simulink model "mainV02_33"  (R2016b)
settings: Solver=FixedStepAuto  StartTime=0.0  StopTime=inf  FixedStep=Ts  MaxStep=0.2  RelTol=1e-2
undefined symbols (not defined in the file): checks, deltae_degrees, deltafl_degrees, deltafr_degrees, deltar_degrees, deltat_1, deltat_2, deltat_3, deltat_4, deltat_5, Earth, F, ft, groundReaction, initialValues, LD, Light, m, MIL, Newton, Raphson, s, sigbuilder_block, Ts, WGS84
libraries: aerolibutil x19, simulink x17, aerolibtransform2 x7, aerolibasang x4, aerolib6dofsys x4, aerolib6dof2 x4, aerolibwind2 x3, aerolibbdyn x3, aerolibconvert2 x3, aerolibconvert x2, vrlib x2, aerolibatmos2 x1
(part 3 of 5)

== system mainV02_33/Sensors (Feedthrough)/Pitot ==
  Environment : Inport  OutDataTypeStr=Bus: envDataBus
  States : Inport  Port=2  OutDataTypeStr=Bus: plantDataBus
  Bus Selector : BusSelector  OutputSignals=V_body
  Bus Selector1 : BusSelector  OutputSignals=windVelocity
  Sum : Sum  Inputs=|+-
  VaeroMeas_body : Outport
  wires:
  Bus Selector/1 -> Sum/1  "<V_body>"
  States/1 -> Bus Selector/1  "plantData"
  Environment/1 -> Bus Selector1/1
  Bus Selector1/1 -> Sum/2  "<windVelocity>"
  Sum/1 -> VaeroMeas_body/1  "VaeroMeas_body"

== system mainV02_33/Sensors (Feedthrough)/Veleta ==
  States : Inport  OutDataTypeStr=Bus: plantDataBus
  Bus Selector : BusSelector  OutputSignals=alpha,beta
  alphaMeas : Outport
  betaMeas : Outport  Port=2
  wires:
  States/1 -> Bus Selector/1  "plantData"
  Bus Selector/1 -> alphaMeas/1  "<alpha>"
  Bus Selector/2 -> betaMeas/1  "<beta>"

== system mainV02_33/Visualization/Airspeed Indicator ==

== system mainV02_33/Visualization/Altimeter ==

== system mainV02_33/Visualization/Artificial Horizon ==

== system mainV02_33/Visualization/Axes to VR Axes ==
  Xe : Inport
  Concatenate : Concatenate  NumInputs=3
  Constant : Constant  Value=1.01
  Demux : Demux  Outputs=3
  Sum : Sum  Inputs=|++
  rad-->deg : Gain  Gain=-1  SaturateOnIntegerOverflow=on  OutDataTypeStr=Inherit: Same as input  ParamDataTypeStr=Inherit: Same as input
  rad-->deg1 : Gain  Gain=-1  SaturateOnIntegerOverflow=on  OutDataTypeStr=Inherit: Same as input  ParamDataTypeStr=Inherit: Same as input
  Xe VR : Outport
  wires:
  Xe/1 -> Demux/1
  Concatenate/1 -> Xe VR/1
  rad-->deg1/1 -> Concatenate/2
  rad-->deg/1 -> Concatenate/1
  Demux/1 -> Concatenate/3
  Demux/2 -> rad-->deg/1
  Constant/1 -> Sum/2
  Demux/3 -> Sum/1
  Sum/1 -> rad-->deg1/1

== system mainV02_33/Visualization/Climb Rate Indicator ==

== system mainV02_33/Visualization/Euler to VR ==
  Euler Angles : Inport
  Axis Angle Vector : Subsystem
  Constant : Constant  Value=pi/2
  Demux : Demux  Outputs=3
  Mux : Mux  Inputs=2
  Mux1 : Mux  Inputs=2
  Mux2 : Mux  Inputs=2
  Quaternion Multiplication (Pitch & Yaw) : aerolibutil/Quaternion Multiplication
  Quaternion Multiplication (Roll) : aerolibutil/Quaternion Multiplication
  Quaternion Normalization : Subsystem
  Quaternion Normalization1 : Subsystem
  Quaternion Normalization2 : Subsystem
  Sum : Sum  Inputs=|++
  Vr Pitch Axes : Constant  Value=[0 0 1]
  Vr Roll Axes : Constant  Value=[1 0 0]
  Vr Yaw Axes : Constant  Value=[0 -1 0]
  Axis Angle : Outport
  wires:
  Quaternion Multiplication (Roll)/1 -> Axis Angle Vector/1(e0)
  Quaternion Multiplication (Pitch & Yaw)/1 -> Quaternion Multiplication (Roll)/2
  Axis Angle Vector/1(e0_norm) -> Axis Angle/1
  Quaternion Normalization/1(e0_norm) -> Quaternion Multiplication (Roll)/1
  Quaternion Normalization2/1(e0_norm) -> Quaternion Multiplication (Pitch & Yaw)/1
  Quaternion Normalization1/1(e0_norm) -> Quaternion Multiplication (Pitch & Yaw)/2
  Mux2/1 -> Quaternion Normalization2/1(e0)
  Mux1/1 -> Quaternion Normalization1/1(e0)
  Mux/1 -> Quaternion Normalization/1(e0)
  Vr Yaw Axes/1 -> Mux2/2
  Demux/2 -> Mux1/1
  Vr Pitch Axes/1 -> Mux1/2
  Demux/1 -> Mux/1
  Vr Roll Axes/1 -> Mux/2
  Euler Angles/1 -> Demux/1
  Sum/1 -> Mux2/1
  Demux/3 -> Sum/1
  Constant/1 -> Sum/2

== system mainV02_33/Visualization/Heading Indicator ==

== system mainV02_33/Visualization/Subsystem ==
  "X_ned " : Inport
  Euler_angles : Inport  Port=2
  V_body : Inport  Port=3
  V_ned : Inport  Port=4
  Angle Conversion : aerolibconvert2/Angle Conversion  IU=rad  OU=deg
  Angle Conversion1 : aerolibconvert2/Angle Conversion  IU=rad  OU=deg
  Climbrate : Selector  IndexMode=Zero-based  InputPortWidth=3  IndexOptions=Index vector (dialog)  Indices=2  OutputSizes=1
  Concatenate : Concatenate
  Dot Product : DotProduct  SaturateOnIntegerOverflow=on  OutDataTypeStr=Inherit: Inherit via internal rule
  Flightpath Angle : Subsystem
  Heading : Selector  IndexMode=Zero-based  InputPortWidth=3  IndexOptions=Index vector (dialog)  Indices=2  OutputSizes=1
  Height : Selector  IndexMode=Zero-based  InputPortWidth=3  IndexOptions=Index vector (dialog)  Indices=2  OutputSizes=1
  Length Conversion : aerolibconvert2/Length Conversion  IU=m  OU=ft
  Roll Angle : Selector  IndexMode=Zero-based  InputPortWidth=3  IndexOptions=Index vector (dialog)  Indices=0  OutputSizes=1
  Velocity Conversion : aerolibconvert/Velocity Conversion  IU=m/s  OU=kts
  Velocity Conversion1 : aerolibconvert/Velocity Conversion  IU=m/s  OU=ft/s
  rad-->deg1 : Gain  Gain=-1  SaturateOnIntegerOverflow=on  OutDataTypeStr=Inherit: Same as input  ParamDataTypeStr=Inherit: Same as input
  rad-->deg2 : Gain  Gain=-1  SaturateOnIntegerOverflow=on  OutDataTypeStr=Inherit: Same as input  ParamDataTypeStr=Inherit: Same as input
  rad-->deg3 : Gain  Gain=60  SaturateOnIntegerOverflow=on  OutDataTypeStr=Inherit: Same as input  ParamDataTypeStr=Inherit: Same as input
  vt : Sqrt  SaturateOnIntegerOverflow=on
  Airspeed (kts) : Outport
  Height (ft) : Outport  Port=2
  Roll Flightpath (deg) : Outport  Port=3
  Climb Rate (ft/min) : Outport  Port=4
  Heading (deg) : Outport  Port=5
  wires:
  Velocity Conversion1/1 -> rad-->deg3/1
  rad-->deg3/1 -> Climb Rate (ft/min)/1
  V_ned/1 -> Flightpath Angle/1(Ve), Climbrate/1
  Flightpath Angle/1(gamma) -> Concatenate/2
  rad-->deg2/1 -> Velocity Conversion1/1
  Length Conversion/1 -> Height (ft)/1
  Angle Conversion1/1 -> Roll Flightpath (deg)/1
  Height/1 -> rad-->deg1/1
  Angle Conversion/1 -> Heading (deg)/1  "Heading"
  Heading/1 -> Angle Conversion/1
  Velocity Conversion/1 -> Airspeed (kts)/1
  Dot Product/1 -> vt/1
  Roll Angle/1 -> Concatenate/1
  V_body/1 -> Dot Product/2, Dot Product/1
  Concatenate/1 -> Angle Conversion1/1
  vt/1 -> Velocity Conversion/1
  Climbrate/1 -> rad-->deg2/1
  rad-->deg1/1 -> Length Conversion/1
  Euler_angles/1 -> Roll Angle/1, Heading/1
  "X_ned "/1 -> Height/1

== system mainV02_33/Environment/Terrain/Reaction ==
  X : Inport
  V : Inport  Port=2
  -D1 : Gain  Gain=-groundReaction.D
  -K2 : Gain  Gain=-groundReaction.K
  Constant3 : Constant  Value=0
  Constant4 : Constant  Value=0
  Constant5 : Constant  Value=0
  Mux1 : Mux  Inputs=3
  Product1 : Product
  Sel5 : Selector  InputPortWidth=3  IndexOptions=Index vector (dialog)  Indices=3  OutputSizes=1
  Sel6 : Selector  InputPortWidth=3  IndexOptions=Index vector (dialog)  Indices=3  OutputSizes=1
  Sqrt1 : Sqrt  SaturateOnIntegerOverflow=on
  Sum4 : Sum  Inputs=|++
  Sum5 : Sum  Inputs=-+
  Switch3 : Switch  Criteria=u2 > Threshold
  Ze2height1 : UnaryMinus
  Ze_dot2height_dot3 : UnaryMinus
  height2d2 : UnaryMinus
  height2d3 : UnaryMinus
  hground_value1 : Constant  Value=initialValues.href  OutDataTypeStr=double
  hground1 : Outport  Unit=m
  F_earth : Outport  Port=2
  wires:
  Ze2height1/1 -> Sum5/2  "alt"
  X/1 -> Sel6/1
  Sel6/1 -> Ze2height1/1
  Sel5/1 -> Ze_dot2height_dot3/1
  hground_value1/1 -> Sum5/1
  Constant3/1 -> Switch3/1
  Switch3/1 -> height2d2/1
  height2d2/1 -> Sqrt1/1  "d"
  -K2/1 -> Sum4/1
  Product1/1 -> height2d3/1
  height2d3/1 -> Mux1/3
  Sum5/1 -> hground1/1, -K2/1, Switch3/3, Switch3/2  "z"
  Sqrt1/1 -> Product1/1
  Ze_dot2height_dot3/1 -> -D1/1  "z_dot"
  -D1/1 -> Sum4/2
  Sum4/1 -> Product1/2
  V/1 -> Sel5/1
  Mux1/1 -> F_earth/1  "F_earth"
  Constant5/1 -> Mux1/2
  Constant4/1 -> Mux1/1

== system mainV02_33/Environment/Terrain/Reaction1 ==
  X : Inport
  V : Inport  Port=2
  -D1 : Gain  Gain=-groundReaction.D
  -K2 : Gain  Gain=-groundReaction.K
  Constant3 : Constant  Value=0
  Constant4 : Constant  Value=0
  Constant5 : Constant  Value=0
  Mux1 : Mux  Inputs=3
  Product1 : Product
  Sel5 : Selector  InputPortWidth=3  IndexOptions=Index vector (dialog)  Indices=3  OutputSizes=1
  Sel6 : Selector  InputPortWidth=3  IndexOptions=Index vector (dialog)  Indices=3  OutputSizes=1
  Sqrt1 : Sqrt  SaturateOnIntegerOverflow=on
  Sum4 : Sum  Inputs=|++
  Sum5 : Sum  Inputs=-+
  Switch3 : Switch  Criteria=u2 > Threshold
  Ze2height1 : UnaryMinus
  Ze_dot2height_dot3 : UnaryMinus
  height2d2 : UnaryMinus
  height2d3 : UnaryMinus
  hground_value1 : Constant  Value=initialValues.href  OutDataTypeStr=double
  hground1 : Outport  Unit=m
  F_earth : Outport  Port=2
  wires:
  Ze2height1/1 -> Sum5/2  "alt"
  X/1 -> Sel6/1
  Sel6/1 -> Ze2height1/1
  Sel5/1 -> Ze_dot2height_dot3/1
  hground_value1/1 -> Sum5/1
  Constant3/1 -> Switch3/1
  Switch3/1 -> height2d2/1
  height2d2/1 -> Sqrt1/1  "d"
  -K2/1 -> Sum4/1
  Product1/1 -> height2d3/1
  height2d3/1 -> Mux1/3
  Sum5/1 -> hground1/1, -K2/1, Switch3/3, Switch3/2  "z"
  Sqrt1/1 -> Product1/1
  Ze_dot2height_dot3/1 -> -D1/1  "z_dot"
  -D1/1 -> Sum4/2
  Sum4/1 -> Product1/2
  V/1 -> Sel5/1
  Mux1/1 -> F_earth/1  "F_earth"
  Constant5/1 -> Mux1/2
  Constant4/1 -> Mux1/1

== system mainV02_33/Environment/Terrain/Reaction2 ==
  X : Inport
  V : Inport  Port=2
  -D1 : Gain  Gain=-groundReaction.D
  -K2 : Gain  Gain=-groundReaction.K
  Constant3 : Constant  Value=0
  Constant4 : Constant  Value=0
  Constant5 : Constant  Value=0
  Mux1 : Mux  Inputs=3
  Product1 : Product
  Sel5 : Selector  InputPortWidth=3  IndexOptions=Index vector (dialog)  Indices=3  OutputSizes=1
  Sel6 : Selector  InputPortWidth=3  IndexOptions=Index vector (dialog)  Indices=3  OutputSizes=1
  Sqrt1 : Sqrt  SaturateOnIntegerOverflow=on
  Sum4 : Sum  Inputs=|++
  Sum5 : Sum  Inputs=-+
  Switch3 : Switch  Criteria=u2 > Threshold
  Ze2height1 : UnaryMinus
  Ze_dot2height_dot3 : UnaryMinus
  height2d2 : UnaryMinus
  height2d3 : UnaryMinus
  hground_value1 : Constant  Value=initialValues.href  OutDataTypeStr=double
  hground1 : Outport  Unit=m
  F_earth : Outport  Port=2
  wires:
  Ze2height1/1 -> Sum5/2  "alt"
  X/1 -> Sel6/1
  Sel6/1 -> Ze2height1/1
  Sel5/1 -> Ze_dot2height_dot3/1
  hground_value1/1 -> Sum5/1
  Constant3/1 -> Switch3/1
  Switch3/1 -> height2d2/1
  height2d2/1 -> Sqrt1/1  "d"
  -K2/1 -> Sum4/1
  Product1/1 -> height2d3/1
  height2d3/1 -> Mux1/3
  Sum5/1 -> hground1/1, -K2/1, Switch3/3, Switch3/2  "z"
  Sqrt1/1 -> Product1/1
  Ze_dot2height_dot3/1 -> -D1/1  "z_dot"
  -D1/1 -> Sum4/2
  Sum4/1 -> Product1/2
  V/1 -> Sel5/1
  Mux1/1 -> F_earth/1  "F_earth"
  Constant5/1 -> Mux1/2
  Constant4/1 -> Mux1/1

== system mainV02_33/FCS/Quad actuator commands/Altitude ==
  Altitude cmd : Inport
  Bias : Bias  Bias=LD.FCS.Quadcopter.Throttle.bias
  dThrottle : Gain  Gain=LD.FCS.Quadcopter.Throttle.dThrottle
  T5 : Outport
  T3 : Outport  Port=2
  T4 : Outport  Port=3
  T2 : Outport  Port=4
  wires:
  Bias/1 -> T5/1, T4/1, T3/1, T2/1
  Altitude cmd/1 -> dThrottle/1
  dThrottle/1 -> Bias/1

== system mainV02_33/FCS/Quad actuator commands/Pitch ==
  Pitch Cmd : Inport
  Constant1 : Constant  Value=LD.Inertia.CG
  Constant2 : Constant  Value=LD.Inertia.CG
  Divide : Product  Inputs=*/
  Product : Product
  Product1 : Product
  Selector : Selector  InputPortWidth=3  IndexOptions=Index vector (dialog)  Indices=1  OutputSizes=1
  Selector1 : Selector  InputPortWidth=3  IndexOptions=Index vector (dialog)  Indices=1  OutputSizes=1
  Sum1 : Sum  Inputs=+-|
  Sum2 : Sum  Inputs=+-|
  dPitch : Gain  Gain=LD.FCS.Quadcopter.Pitch.dPitch
  "motor2 position " : Constant  Value=LD.Propulsion.motor2.Position
  motor2 position 1 : Constant  Value=LD.Propulsion.motor3.Position
  T5 : Outport
  T3 : Outport  Port=2
  T2 : Outport  Port=3
  T4 : Outport  Port=4
  wires:
  Pitch Cmd/1 -> dPitch/1
  Product/1 -> T3/1
  dPitch/1 -> T5/1, Product1/1, Product/1, T2/1
  Constant1/1 -> Sum1/2
  "motor2 position "/1 -> Sum1/1
  Sum1/1 -> Selector/1  "arm"
  Constant2/1 -> Sum2/2
  motor2 position 1/1 -> Sum2/1
  Sum2/1 -> Selector1/1  "arm"
  Selector/1 -> Divide/1
  Selector1/1 -> Divide/2
  Product1/1 -> T4/1
  [Gain] -> Product/2
  [Gain] -> Product1/2
  Divide/1 -> [Gain]

== system mainV02_33/FCS/Quad actuator commands/Roll ==
  Roll Cmd : Inport
  Gain : Gain  Gain=-1
  Gain1 : Gain  Gain=-1
  dRoll : Gain  Gain=LD.FCS.Quadcopter.Roll.dRoll
  T4 : Outport
  T2 : Outport  Port=2
  T5 : Outport  Port=3
  T3 : Outport  Port=4
  wires:
  Gain/1 -> T2/1
  dRoll/1 -> Gain1/1, Gain/1, T4/1, T5/1
  Roll Cmd/1 -> dRoll/1
  Gain1/1 -> T3/1

== system mainV02_33/FCS/Quad actuator commands/Yaw ==
  Yaw Cmd : Inport
  Gain : Gain  Gain=-1
  Gain1 : Gain  Gain=-1
  dYaw : Gain  Gain=LD.FCS.Quadcopter.Yaw.dYaw
  T5 : Outport
  T4 : Outport  Port=2
  T3 : Outport  Port=3
  T2 : Outport  Port=4
  wires:
  Yaw Cmd/1 -> dYaw/1
  dYaw/1 -> Gain1/1, T4/1, T2/1, Gain/1
  Gain1/1 -> T5/1
  Gain/1 -> T3/1

== system mainV02_33/LIBIS Plant/Aerodynamics/CD ==
  prelook-ups : Inport
  plantData : Inport  Port=2
  actuators : Inport  Port=3
  Add : Sum  Inputs=+++++++
  Bus Selector : BusSelector  OutputSignals=alpha,alpha_dot,Omega_body.q
  Bus Selector1 : BusSelector  OutputSignals=alpha,beta,alt,xcg,deltae,deltar,deltafr,deltafl
  Bus Selector2 : BusSelector  OutputSignals=deltae,deltafr,deltafl
  CD0 : Interpolation_n-D  NumberOfTableDimensions=8  Table=LD.Stability.CD0  ExtrapMethod=Clip  DiagnosticForOutOfRangeInput=Warning  RequireIndexFractionAsBus=on  ValidIndexMayReachLast=on  InternalRulePriority=Speed
      settings: InputPortMap=u0,u1,u2,u3,u4,u5,u6,u7
  CDalpha : Interpolation_n-D  NumberOfTableDimensions=8  Table=LD.Stability.CDalpha  ExtrapMethod=Clip  DiagnosticForOutOfRangeInput=Warning  RequireIndexFractionAsBus=on  ValidIndexMayReachLast=on  InternalRulePriority=Speed
      settings: InputPortMap=u0,u1,u2,u3,u4,u5,u6,u7
  CDalpha_dot : Interpolation_n-D  NumberOfTableDimensions=8  Table=LD.Stability.CDalpha_dot  ExtrapMethod=Clip  RequireIndexFractionAsBus=on  ValidIndexMayReachLast=on  InternalRulePriority=Speed
      settings: InputPortMap=u0,u1,u2,u3,u4,u5,u6,u7
  CDdeltae : Interpolation_n-D  NumberOfTableDimensions=8  Table=LD.Stability.CDdeltae  ExtrapMethod=Clip  RequireIndexFractionAsBus=on  ValidIndexMayReachLast=on  InternalRulePriority=Speed
      settings: InputPortMap=u0,u1,u2,u3,u4,u5,u6,u7
  CDdeltafr : Interpolation_n-D  NumberOfTableDimensions=8  Table=LD.Stability.CDdeltafr  ExtrapMethod=Clip  RequireIndexFractionAsBus=on  ValidIndexMayReachLast=on  InternalRulePriority=Speed
      settings: InputPortMap=u0,u1,u2,u3,u4,u5,u6,u7
  CDdeltafrl : Interpolation_n-D  NumberOfTableDimensions=8  Table=LD.Stability.CDdeltafl  ExtrapMethod=Clip  RequireIndexFractionAsBus=on  ValidIndexMayReachLast=on  InternalRulePriority=Speed
      settings: InputPortMap=u0,u1,u2,u3,u4,u5,u6,u7
  CDq : Interpolation_n-D  NumberOfTableDimensions=8  Table=LD.Stability.CDq  ExtrapMethod=Clip  RequireIndexFractionAsBus=on  ValidIndexMayReachLast=on  InternalRulePriority=Speed
      settings: InputPortMap=u0,u1,u2,u3,u4,u5,u6,u7
  Product{,1..5} (6 alike) : Product
  CD : Outport
  wires:
  prelook-ups/1 -> Bus Selector1/1
  CD0/1 -> Add/1
  Add/1 -> CD/1
  plantData/1 -> Bus Selector/1
  actuators/1 -> Bus Selector2/1
  Product/1 -> Add/2
  Bus Selector/1 -> Product/2  "<alpha>"
  Bus Selector2/1 -> Product3/2  "<deltae>"
  CDdeltae/1 -> Product3/1
  Product3/1 -> Add/5
  Product2/1 -> Add/4
  Product1/1 -> Add/3
  CDalpha_dot/1 -> Product1/1
  CDq/1 -> Product2/1
  Bus Selector/3 -> Product2/2  "<q>"
  Bus Selector/2 -> Product1/2  "<alpha_dot>"
  Bus Selector1/8 -> CD0/8, CDalpha/8, CDq/8, CDdeltafrl/8, CDdeltafr/8, CDdeltae/8, CDalpha_dot/8  "<deltafl>"
  Bus Selector1/7 -> CD0/7, CDalpha/7, CDq/7, CDdeltafrl/7, CDdeltafr/7, CDdeltae/7, CDalpha_dot/7  "<deltafr>"
  Bus Selector1/6 -> CD0/6, CDalpha/6, CDq/6, CDdeltafrl/6, CDdeltafr/6, CDdeltae/6, CDalpha_dot/6  "<deltar>"
  Bus Selector1/5 -> CD0/5, CDalpha/5, CDq/5, CDdeltafrl/5, CDdeltafr/5, CDdeltae/5, CDalpha_dot/5  "<deltae>"
  Bus Selector1/3 -> CD0/3, CDalpha/3, CDq/3, CDdeltafrl/3, CDdeltafr/3, CDdeltae/3, CDalpha_dot/3  "<alt>"
  Bus Selector1/4 -> CD0/4, CDalpha/4, CDq/4, CDdeltafrl/4, CDdeltafr/4, CDdeltae/4, CDalpha_dot/4  "<xcg>"
  Bus Selector1/1 -> CD0/1, CDalpha/1, CDdeltafrl/1, CDdeltafr/1, CDdeltae/1, CDq/1, CDalpha_dot/1  "<alpha>"
  Bus Selector2/3 -> Product5/2  "<deltafl>"
  CDdeltafrl/1 -> Product5/1
  Product5/1 -> Add/7
  Product4/1 -> Add/6
  CDdeltafr/1 -> Product4/1
  Bus Selector2/2 -> Product4/2  "<deltafr>"
  Bus Selector1/2 -> CD0/2, CDdeltafrl/2, CDdeltafr/2, CDdeltae/2, CDq/2, CDalpha_dot/2, CDalpha/2  "<beta>"
  CDalpha/1 -> Product/1

== system mainV02_33/LIBIS Plant/Aerodynamics/CL ==
  prelook-ups : Inport
  plantData : Inport  Port=2
  actuators : Inport  Port=3
  Add1 : Sum  Inputs=+++++++
  Bus Selector2 : BusSelector  OutputSignals=alpha,alpha_dot,Omega_body.q
  Bus Selector4 : BusSelector  OutputSignals=alpha,beta,alt,xcg,deltae,deltar,deltafr,deltafl
  Bus Selector5 : BusSelector  OutputSignals=deltae,deltafr,deltafl
  CL0 : Interpolation_n-D  NumberOfTableDimensions=8  Table=LD.Stability.CL0  RequireIndexFractionAsBus=on  InternalRulePriority=Speed
      settings: InputPortMap=u0,u1,u2,u3,u4,u5,u6,u7
  CLalpha : Interpolation_n-D  NumberOfTableDimensions=8  Table=LD.Stability.CLalpha  ExtrapMethod=Clip  DiagnosticForOutOfRangeInput=Warning  RequireIndexFractionAsBus=on  ValidIndexMayReachLast=on  InternalRulePriority=Speed
      settings: InputPortMap=u0,u1,u2,u3,u4,u5,u6,u7
  CLalpha_dot : Interpolation_n-D  NumberOfTableDimensions=8  Table=LD.Stability.CLalpha_dot  ExtrapMethod=Clip  RequireIndexFractionAsBus=on  ValidIndexMayReachLast=on  InternalRulePriority=Speed
      settings: InputPortMap=u0,u1,u2,u3,u4,u5,u6,u7
  CLdeltae : Interpolation_n-D  NumberOfTableDimensions=8  Table=LD.Stability.CLdeltae  ExtrapMethod=Clip  RequireIndexFractionAsBus=on  ValidIndexMayReachLast=on  InternalRulePriority=Speed
      settings: InputPortMap=u0,u1,u2,u3,u4,u5,u6,u7
  CLdeltafr : Interpolation_n-D  NumberOfTableDimensions=8  Table=LD.Stability.CLdeltafr  ExtrapMethod=Clip  RequireIndexFractionAsBus=on  ValidIndexMayReachLast=on  InternalRulePriority=Speed
      settings: InputPortMap=u0,u1,u2,u3,u4,u5,u6,u7
  CLdeltafrl : Interpolation_n-D  NumberOfTableDimensions=8  Table=LD.Stability.CLdeltafl  ExtrapMethod=Clip  RequireIndexFractionAsBus=on  ValidIndexMayReachLast=on  InternalRulePriority=Speed
      settings: InputPortMap=u0,u1,u2,u3,u4,u5,u6,u7
  CLq : Interpolation_n-D  NumberOfTableDimensions=8  Table=LD.Stability.CLq  ExtrapMethod=Clip  RequireIndexFractionAsBus=on  ValidIndexMayReachLast=on  InternalRulePriority=Speed
      settings: InputPortMap=u0,u1,u2,u3,u4,u5,u6,u7
  Product{6..11} (6 alike) : Product
  CL : Outport
  wires:
  prelook-ups/1 -> Bus Selector4/1
  CL0/1 -> Add1/1
  Add1/1 -> CL/1
  plantData/1 -> Bus Selector2/1
  actuators/1 -> Bus Selector5/1
  Product6/1 -> Add1/2
  Bus Selector2/1 -> Product6/2  "<alpha>"
  Bus Selector5/1 -> Product9/2  "<deltae>"
  CLdeltae/1 -> Product9/1
  Product9/1 -> Add1/5
  Product8/1 -> Add1/4
  Product7/1 -> Add1/3
  CLalpha_dot/1 -> Product7/1
  CLq/1 -> Product8/1
  Bus Selector2/3 -> Product8/2  "<q>"
  Bus Selector2/2 -> Product7/2  "<alpha_dot>"
  Bus Selector4/8 -> CL0/8, CLalpha/8, CLq/8, CLdeltafrl/8, CLdeltafr/8, CLdeltae/8, CLalpha_dot/8  "<deltafl>"
  Bus Selector4/7 -> CL0/7, CLalpha/7, CLq/7, CLdeltafrl/7, CLdeltafr/7, CLdeltae/7, CLalpha_dot/7  "<deltafr>"
  Bus Selector4/6 -> CL0/6, CLalpha/6, CLq/6, CLdeltafrl/6, CLdeltafr/6, CLdeltae/6, CLalpha_dot/6  "<deltar>"
  Bus Selector4/5 -> CL0/5, CLalpha/5, CLq/5, CLdeltafrl/5, CLdeltafr/5, CLdeltae/5, CLalpha_dot/5  "<deltae>"
  Bus Selector4/3 -> CL0/3, CLalpha/3, CLq/3, CLdeltafrl/3, CLdeltafr/3, CLdeltae/3, CLalpha_dot/3  "<alt>"
  Bus Selector4/4 -> CL0/4, CLalpha/4, CLq/4, CLdeltafrl/4, CLdeltafr/4, CLdeltae/4, CLalpha_dot/4  "<xcg>"
  Bus Selector4/1 -> CL0/1, CLalpha/1, CLdeltafrl/1, CLdeltafr/1, CLdeltae/1, CLq/1, CLalpha_dot/1  "<alpha>"
  Bus Selector5/3 -> Product11/2  "<deltafl>"
  CLdeltafrl/1 -> Product11/1
  Product11/1 -> Add1/7
  Product10/1 -> Add1/6
  CLdeltafr/1 -> Product10/1
  Bus Selector5/2 -> Product10/2  "<deltafr>"
  Bus Selector4/2 -> CL0/2, CLdeltafrl/2, CLdeltafr/2, CLdeltae/2, CLq/2, CLalpha_dot/2, CLalpha/2  "<beta>"
  CLalpha/1 -> Product6/1

== system mainV02_33/LIBIS Plant/Aerodynamics/CY ==
  prelook-ups : Inport
  plantData : Inport  Port=2
  actuators : Inport  Port=3
  Add : Sum  Inputs=++++++
  Bus Selector : BusSelector  OutputSignals=beta,Omega_body.p,Omega_body.r
  Bus Selector1 : BusSelector  OutputSignals=alpha,beta,alt,xcg,deltae,deltar,deltafr,deltafl
  Bus Selector2 : BusSelector  OutputSignals=deltar,deltafr,deltafl
  CYbeta : Interpolation_n-D  NumberOfTableDimensions=8  Table=LD.Stability.CYbeta  ExtrapMethod=Clip  RequireIndexFractionAsBus=on  ValidIndexMayReachLast=on  InternalRulePriority=Speed
      settings: InputPortMap=u0,u1,u2,u3,u4,u5,u6,u7
  CYdeltafl : Interpolation_n-D  NumberOfTableDimensions=8  Table=LD.Stability.CYdeltafl  ExtrapMethod=Clip  RequireIndexFractionAsBus=on  ValidIndexMayReachLast=on  InternalRulePriority=Speed
      settings: InputPortMap=u0,u1,u2,u3,u4,u5,u6,u7
  CYdeltafr : Interpolation_n-D  NumberOfTableDimensions=8  Table=LD.Stability.CYdeltafr  ExtrapMethod=Clip  RequireIndexFractionAsBus=on  ValidIndexMayReachLast=on  InternalRulePriority=Speed
      settings: InputPortMap=u0,u1,u2,u3,u4,u5,u6,u7
  "CYdeltar " : Interpolation_n-D  NumberOfTableDimensions=8  Table=LD.Stability.CYdeltar  ExtrapMethod=Clip  RequireIndexFractionAsBus=on  ValidIndexMayReachLast=on  InternalRulePriority=Speed
      settings: InputPortMap=u0,u1,u2,u3,u4,u5,u6,u7
  CYp : Interpolation_n-D  NumberOfTableDimensions=8  Table=LD.Stability.CYp  ExtrapMethod=Clip  RequireIndexFractionAsBus=on  ValidIndexMayReachLast=on  InternalRulePriority=Speed
      settings: InputPortMap=u0,u1,u2,u3,u4,u5,u6,u7
  CYr : Interpolation_n-D  NumberOfTableDimensions=8  Table=LD.Stability.CYr  ExtrapMethod=Clip  RequireIndexFractionAsBus=on  ValidIndexMayReachLast=on  InternalRulePriority=Speed
      settings: InputPortMap=u0,u1,u2,u3,u4,u5,u6,u7
  Product{,1..5} (6 alike) : Product
  CY : Outport
  wires:
  Bus Selector1/8 -> CYbeta/8, CYr/8, "CYdeltar "/8, CYdeltafl/8, CYdeltafr/8, CYp/8  "<deltafl>"
  Bus Selector1/7 -> CYbeta/7, CYr/7, "CYdeltar "/7, CYdeltafl/7, CYdeltafr/7, CYp/7  "<deltafr>"
  Bus Selector1/6 -> CYbeta/6, CYr/6, "CYdeltar "/6, CYdeltafl/6, CYdeltafr/6, CYp/6  "<deltar>"
  prelook-ups/1 -> Bus Selector1/1
  Bus Selector1/5 -> CYbeta/5, CYr/5, "CYdeltar "/5, CYdeltafl/5, CYdeltafr/5, CYp/5  "<deltae>"
  Bus Selector1/3 -> CYbeta/3, CYr/3, "CYdeltar "/3, CYdeltafl/3, CYdeltafr/3, CYp/3  "<alt>"
  Bus Selector1/4 -> CYbeta/4, CYr/4, "CYdeltar "/4, CYdeltafl/4, CYdeltafr/4, CYp/4  "<xcg>"
  Bus Selector1/1 -> CYbeta/1, CYdeltafl/1, CYdeltafr/1, "CYdeltar "/1, CYr/1, CYp/1  "<alpha>"
  Add/1 -> CY/1
  plantData/1 -> Bus Selector/1
  actuators/1 -> Bus Selector2/1
  CYbeta/1 -> Product/1
  Product/1 -> Add/1
  Bus Selector/1 -> Product/2  "<beta>"
  Bus Selector2/1 -> Product3/2  "<deltar>"
  "CYdeltar "/1 -> Product3/1
  Product3/1 -> Add/4
  Product2/1 -> Add/3
  Product1/1 -> Add/2
  CYp/1 -> Product1/1
  CYr/1 -> Product2/1
  Bus Selector/3 -> Product2/2  "<r>"
  Bus Selector/2 -> Product1/2  "<p>"
  CYdeltafl/1 -> Product5/1
  Product5/1 -> Add/6
  Product4/1 -> Add/5
  CYdeltafr/1 -> Product4/1
  Bus Selector2/2 -> Product4/2  "<deltafr>"
  Bus Selector2/3 -> Product5/2  "<deltafl>"
  Bus Selector1/2 -> CYdeltafl/2, CYdeltafr/2, "CYdeltar "/2, CYr/2, CYp/2, CYbeta/2  "<beta>"

== system mainV02_33/LIBIS Plant/Aerodynamics/Cl ==
  prelook-ups1 : Inport
  plantData : Inport  Port=2
  actuators : Inport  Port=3
  Add1 : Sum  Inputs=++++++
  Bus Selector3 : BusSelector  OutputSignals=beta,Omega_body.p,Omega_body.r
  Bus Selector4 : BusSelector  OutputSignals=alpha,beta,alt,xcg,deltae,deltar,deltafr,deltafl
  Bus Selector5 : BusSelector  OutputSignals=deltar,deltafr,deltafl
  Clbeta : Interpolation_n-D  NumberOfTableDimensions=8  Table=LD.Stability.Clbeta  ExtrapMethod=Clip  RequireIndexFractionAsBus=on  ValidIndexMayReachLast=on  InternalRulePriority=Speed
      settings: InputPortMap=u0,u1,u2,u3,u4,u5,u6,u7
  Cldeltafl : Interpolation_n-D  NumberOfTableDimensions=8  Table=LD.Stability.Cldeltafl  ExtrapMethod=Clip  RequireIndexFractionAsBus=on  ValidIndexMayReachLast=on  InternalRulePriority=Speed
      settings: InputPortMap=u0,u1,u2,u3,u4,u5,u6,u7
  Cldeltafr : Interpolation_n-D  NumberOfTableDimensions=8  Table=LD.Stability.Cldeltafr  ExtrapMethod=Clip  RequireIndexFractionAsBus=on  ValidIndexMayReachLast=on  InternalRulePriority=Speed
      settings: InputPortMap=u0,u1,u2,u3,u4,u5,u6,u7
  "Cldeltar " : Interpolation_n-D  NumberOfTableDimensions=8  Table=LD.Stability.Cldeltar  ExtrapMethod=Clip  RequireIndexFractionAsBus=on  ValidIndexMayReachLast=on  InternalRulePriority=Speed
      settings: InputPortMap=u0,u1,u2,u3,u4,u5,u6,u7
  Clp : Interpolation_n-D  NumberOfTableDimensions=8  Table=LD.Stability.Clp  ExtrapMethod=Clip  RequireIndexFractionAsBus=on  ValidIndexMayReachLast=on  InternalRulePriority=Speed
      settings: InputPortMap=u0,u1,u2,u3,u4,u5,u6,u7
  Clr : Interpolation_n-D  NumberOfTableDimensions=8  Table=LD.Stability.Clr  ExtrapMethod=Clip  RequireIndexFractionAsBus=on  ValidIndexMayReachLast=on  InternalRulePriority=Speed
      settings: InputPortMap=u0,u1,u2,u3,u4,u5,u6,u7
  Product{6..11} (6 alike) : Product
  Cl : Outport
  wires:
  Bus Selector4/8 -> Clbeta/8, Clr/8, "Cldeltar "/8, Cldeltafl/8, Cldeltafr/8, Clp/8  "<deltafl>"
  Bus Selector4/7 -> Clbeta/7, Clr/7, "Cldeltar "/7, Cldeltafl/7, Cldeltafr/7, Clp/7  "<deltafr>"
  Bus Selector4/6 -> Clbeta/6, Clr/6, "Cldeltar "/6, Cldeltafl/6, Cldeltafr/6, Clp/6  "<deltar>"
  prelook-ups1/1 -> Bus Selector4/1
  Bus Selector4/5 -> Clbeta/5, Clr/5, "Cldeltar "/5, Cldeltafl/5, Cldeltafr/5, Clp/5  "<deltae>"
  Bus Selector4/3 -> Clbeta/3, Clr/3, "Cldeltar "/3, Cldeltafl/3, Cldeltafr/3, Clp/3  "<alt>"
  Bus Selector4/4 -> Clbeta/4, Clr/4, "Cldeltar "/4, Cldeltafl/4, Cldeltafr/4, Clp/4  "<xcg>"
  Bus Selector4/1 -> Clbeta/1, Cldeltafl/1, Cldeltafr/1, "Cldeltar "/1, Clr/1, Clp/1  "<alpha>"
  Add1/1 -> Cl/1
  plantData/1 -> Bus Selector3/1
  actuators/1 -> Bus Selector5/1
  Clbeta/1 -> Product6/1
  Product6/1 -> Add1/1
  Bus Selector3/1 -> Product6/2  "<beta>"
  Bus Selector5/1 -> Product9/2  "<deltar>"
  "Cldeltar "/1 -> Product9/1
  Product9/1 -> Add1/4
  Product8/1 -> Add1/3
  Product7/1 -> Add1/2
  Clp/1 -> Product7/1
  Clr/1 -> Product8/1
  Bus Selector3/3 -> Product8/2  "<r>"
  Bus Selector3/2 -> Product7/2  "<p>"
  Cldeltafl/1 -> Product11/1
  Product11/1 -> Add1/6
  Product10/1 -> Add1/5
  Cldeltafr/1 -> Product10/1
  Bus Selector5/2 -> Product10/2  "<deltafr>"
  Bus Selector5/3 -> Product11/2  "<deltafl>"
  Bus Selector4/2 -> Cldeltafl/2, Cldeltafr/2, "Cldeltar "/2, Clr/2, Clp/2, Clbeta/2  "<beta>"

== system mainV02_33/LIBIS Plant/Aerodynamics/Cm ==
  prelook-ups : Inport
  plantData : Inport  Port=2
  actuators : Inport  Port=3
  Add2 : Sum  Inputs=+++++++
  Bus Selector2 : BusSelector  OutputSignals=alpha,alpha_dot,Omega_body.q
  Bus Selector4 : BusSelector  OutputSignals=alpha,beta,alt,xcg,deltae,deltar,deltafr,deltafl
  Bus Selector5 : BusSelector  OutputSignals=deltae,deltafr,deltafl
  Cm0 : Interpolation_n-D  NumberOfTableDimensions=8  Table=LD.Stability.Cm0  RequireIndexFractionAsBus=on  InternalRulePriority=Speed
      settings: InputPortMap=u0,u1,u2,u3,u4,u5,u6,u7
  Cmalpha : Interpolation_n-D  NumberOfTableDimensions=8  Table=LD.Stability.Cmalpha  ExtrapMethod=Clip  RequireIndexFractionAsBus=on  ValidIndexMayReachLast=on  InternalRulePriority=Speed
      settings: InputPortMap=u0,u1,u2,u3,u4,u5,u6,u7
  Cmalpha_dot : Interpolation_n-D  NumberOfTableDimensions=8  Table=LD.Stability.Cmalpha_dot  ExtrapMethod=Clip  RequireIndexFractionAsBus=on  ValidIndexMayReachLast=on  InternalRulePriority=Speed
      settings: InputPortMap=u0,u1,u2,u3,u4,u5,u6,u7
  Cmdeltae : Interpolation_n-D  NumberOfTableDimensions=8  Table=LD.Stability.Cmdeltae  ExtrapMethod=Clip  RequireIndexFractionAsBus=on  ValidIndexMayReachLast=on  InternalRulePriority=Speed
      settings: InputPortMap=u0,u1,u2,u3,u4,u5,u6,u7
  Cmdeltafl : Interpolation_n-D  NumberOfTableDimensions=8  Table=LD.Stability.CLdeltafl  ExtrapMethod=Clip  RequireIndexFractionAsBus=on  ValidIndexMayReachLast=on  InternalRulePriority=Speed
      settings: InputPortMap=u0,u1,u2,u3,u4,u5,u6,u7
  Cmdeltafr : Interpolation_n-D  NumberOfTableDimensions=8  Table=LD.Stability.Cmdeltafr  ExtrapMethod=Clip  RequireIndexFractionAsBus=on  ValidIndexMayReachLast=on  InternalRulePriority=Speed
      settings: InputPortMap=u0,u1,u2,u3,u4,u5,u6,u7
  Cmq : Interpolation_n-D  NumberOfTableDimensions=8  Table=LD.Stability.Cmq  ExtrapMethod=Clip  RequireIndexFractionAsBus=on  ValidIndexMayReachLast=on  InternalRulePriority=Speed
      settings: InputPortMap=u0,u1,u2,u3,u4,u5,u6,u7
  Product{6..11} (6 alike) : Product
  Cm : Outport
  wires:
  prelook-ups/1 -> Bus Selector4/1
  Cm0/1 -> Add2/1
  Add2/1 -> Cm/1
  plantData/1 -> Bus Selector2/1
  actuators/1 -> Bus Selector5/1
  Product6/1 -> Add2/2
  Bus Selector2/1 -> Product6/2  "<alpha>"
  Bus Selector5/1 -> Product9/2  "<deltae>"
  Cmdeltae/1 -> Product9/1
  Product9/1 -> Add2/5
  Product8/1 -> Add2/4
  Product7/1 -> Add2/3
  Cmalpha_dot/1 -> Product7/1
  Cmq/1 -> Product8/1
  Bus Selector2/3 -> Product8/2  "<q>"
  Bus Selector2/2 -> Product7/2  "<alpha_dot>"
  Bus Selector4/8 -> Cm0/8, Cmalpha/8, Cmq/8, Cmdeltafl/8, Cmdeltafr/8, Cmdeltae/8, Cmalpha_dot/8  "<deltafl>"
  Bus Selector4/7 -> Cm0/7, Cmalpha/7, Cmq/7, Cmdeltafl/7, Cmdeltafr/7, Cmdeltae/7, Cmalpha_dot/7  "<deltafr>"
  Bus Selector4/6 -> Cm0/6, Cmalpha/6, Cmq/6, Cmdeltafl/6, Cmdeltafr/6, Cmdeltae/6, Cmalpha_dot/6  "<deltar>"
  Bus Selector4/5 -> Cm0/5, Cmalpha/5, Cmq/5, Cmdeltafl/5, Cmdeltafr/5, Cmdeltae/5, Cmalpha_dot/5  "<deltae>"
  Bus Selector4/3 -> Cm0/3, Cmalpha/3, Cmq/3, Cmdeltafl/3, Cmdeltafr/3, Cmdeltae/3, Cmalpha_dot/3  "<alt>"
  Bus Selector4/4 -> Cm0/4, Cmalpha/4, Cmq/4, Cmdeltafl/4, Cmdeltafr/4, Cmdeltae/4, Cmalpha_dot/4  "<xcg>"
  Bus Selector4/1 -> Cm0/1, Cmalpha/1, Cmdeltafl/1, Cmdeltafr/1, Cmdeltae/1, Cmq/1, Cmalpha_dot/1  "<alpha>"
  Bus Selector5/3 -> Product11/2  "<deltafl>"
  Cmdeltafl/1 -> Product11/1
  Product11/1 -> Add2/7
  Product10/1 -> Add2/6
  Cmdeltafr/1 -> Product10/1
  Bus Selector5/2 -> Product10/2  "<deltafr>"
  Bus Selector4/2 -> Cm0/2, Cmdeltafl/2, Cmdeltafr/2, Cmdeltae/2, Cmq/2, Cmalpha_dot/2, Cmalpha/2  "<beta>"
  Cmalpha/1 -> Product6/1

== system mainV02_33/LIBIS Plant/Aerodynamics/Cn ==
  prelook-ups : Inport
  plantData : Inport  Port=2
  actuators : Inport  Port=3
  Add1 : Sum  Inputs=++++++
  Bus Selector3 : BusSelector  OutputSignals=beta,Omega_body.p,Omega_body.r
  Bus Selector4 : BusSelector  OutputSignals=alpha,beta,alt,xcg,deltae,deltar,deltafr,deltafl
  Bus Selector5 : BusSelector  OutputSignals=deltar,deltafr,deltafl
  Cnbeta : Interpolation_n-D  NumberOfTableDimensions=8  Table=LD.Stability.Cnbeta  ExtrapMethod=Clip  RequireIndexFractionAsBus=on  ValidIndexMayReachLast=on  InternalRulePriority=Speed
      settings: InputPortMap=u0,u1,u2,u3,u4,u5,u6,u7
  Cndeltafl : Interpolation_n-D  NumberOfTableDimensions=8  Table=LD.Stability.Cndeltafl  ExtrapMethod=Clip  RequireIndexFractionAsBus=on  ValidIndexMayReachLast=on  InternalRulePriority=Speed
      settings: InputPortMap=u0,u1,u2,u3,u4,u5,u6,u7
  Cndeltafr : Interpolation_n-D  NumberOfTableDimensions=8  Table=LD.Stability.Cndeltafr  ExtrapMethod=Clip  RequireIndexFractionAsBus=on  ValidIndexMayReachLast=on  InternalRulePriority=Speed
      settings: InputPortMap=u0,u1,u2,u3,u4,u5,u6,u7
  "Cndeltar " : Interpolation_n-D  NumberOfTableDimensions=8  Table=LD.Stability.Cndeltar  ExtrapMethod=Clip  RequireIndexFractionAsBus=on  ValidIndexMayReachLast=on  InternalRulePriority=Speed
      settings: InputPortMap=u0,u1,u2,u3,u4,u5,u6,u7
  Cnp : Interpolation_n-D  NumberOfTableDimensions=8  Table=LD.Stability.Cnp  ExtrapMethod=Clip  RequireIndexFractionAsBus=on  ValidIndexMayReachLast=on  InternalRulePriority=Speed
      settings: InputPortMap=u0,u1,u2,u3,u4,u5,u6,u7
  Cnr : Interpolation_n-D  NumberOfTableDimensions=8  Table=LD.Stability.Cnr  ExtrapMethod=Clip  RequireIndexFractionAsBus=on  ValidIndexMayReachLast=on  InternalRulePriority=Speed
      settings: InputPortMap=u0,u1,u2,u3,u4,u5,u6,u7
  Product{6..11} (6 alike) : Product
  Cn : Outport
  wires:
  Bus Selector4/8 -> Cnbeta/8, Cnr/8, "Cndeltar "/8, Cndeltafl/8, Cndeltafr/8, Cnp/8  "<deltafl>"
  Bus Selector4/7 -> Cnbeta/7, Cnr/7, "Cndeltar "/7, Cndeltafl/7, Cndeltafr/7, Cnp/7  "<deltafr>"
  Bus Selector4/6 -> Cnbeta/6, Cnr/6, "Cndeltar "/6, Cndeltafl/6, Cndeltafr/6, Cnp/6  "<deltar>"
  prelook-ups/1 -> Bus Selector4/1
  Bus Selector4/5 -> Cnbeta/5, Cnr/5, "Cndeltar "/5, Cndeltafl/5, Cndeltafr/5, Cnp/5  "<deltae>"
  Bus Selector4/3 -> Cnbeta/3, Cnr/3, "Cndeltar "/3, Cndeltafl/3, Cndeltafr/3, Cnp/3  "<alt>"
  Bus Selector4/4 -> Cnbeta/4, Cnr/4, "Cndeltar "/4, Cndeltafl/4, Cndeltafr/4, Cnp/4  "<xcg>"
  Bus Selector4/1 -> Cnbeta/1, Cndeltafl/1, Cndeltafr/1, "Cndeltar "/1, Cnr/1, Cnp/1  "<alpha>"
  Add1/1 -> Cn/1
  plantData/1 -> Bus Selector3/1
  actuators/1 -> Bus Selector5/1
  Cnbeta/1 -> Product6/1
  Product6/1 -> Add1/1
  Bus Selector3/1 -> Product6/2  "<beta>"
  Bus Selector5/1 -> Product9/2  "<deltar>"
  "Cndeltar "/1 -> Product9/1
  Product9/1 -> Add1/4
  Product8/1 -> Add1/3
  Product7/1 -> Add1/2
  Cnp/1 -> Product7/1
  Cnr/1 -> Product8/1
  Bus Selector3/3 -> Product8/2  "<r>"
  Bus Selector3/2 -> Product7/2  "<p>"
  Cndeltafl/1 -> Product11/1
  Product11/1 -> Add1/6
  Product10/1 -> Add1/5
  Cndeltafr/1 -> Product10/1
  Bus Selector5/2 -> Product10/2  "<deltafr>"
  Bus Selector5/3 -> Product11/2  "<deltafl>"
  Bus Selector4/2 -> Cndeltafl/2, Cndeltafr/2, "Cndeltar "/2, Cnr/2, Cnp/2, Cnbeta/2  "<beta>"

== system mainV02_33/LIBIS Plant/Propulsion/8S 25C Battery ==
  note: ZIPPY Compact 5800mAh 8S 25C Lipo Pack
      |
      | Spec.
      | Capacity: 5800mAh
      | Voltage: 8S1P / 8 Cell / 29.6V
      | Discharge: 25C Constant / 35C Burst
      | Weight: 1025g (including wire, plug & case)
      | Dimensions: 167x46x64mm
      | Balance Plug: JST-XH
      | Discharge Plug: 5.5mm Bullet
  note: ZIPPY Compact 5800mAh 8S 25C Lipo Pack
      |
      | SKU
      | ZC.5800.8S.25
      | Weight(g):
      | 1020.00
      | Length:
      | 161.00
      | Width
      | 46.00
      | Height
      | 73.00
      | Capacity (mAh):
      | 5800.00
      | Discharge(c):
      | 25.00
      | Length-A(mm)
      | 167.00
      | Height-B(mm)
      | 46.00
      | Width-C(mm):
      | 64.00
      | Unit Weight (g):
      | 1020
      | Max Charge Rate(C)
      | 5.00
      | Watt Hour
      | 171.00
  note: Batería escogida: 8S 29.6V
  Battery_Capacity : Constant  Value=5.8
  Battery_Voltage : Constant  Value=29.6
  Max_discharge_rate : Constant  Value=145
  profundidad_descarga : Constant  Value=0.95
  rendimiento_bateria : Constant  Value=0.98
  C_battery : Outport  Unit=A*h
  deep_discharge_battery : Outport  Port=2  Unit=1
  V_battery : Outport  Port=3  Unit=V
  eta_battery : Outport  Port=4  Unit=1
  max_discharge_rate : Outport  Port=5  Unit=A*h
  wires:
  Battery_Voltage/1 -> V_battery/1
  Battery_Capacity/1 -> C_battery/1
  profundidad_descarga/1 -> deep_discharge_battery/1
  rendimiento_bateria/1 -> eta_battery/1
  Max_discharge_rate/1 -> max_discharge_rate/1

== system mainV02_33/LIBIS Plant/Propulsion/Variant_Motor_1 ==
  note: 1) Add Subsystem or Model blocks as valid variant choices.
      | 2) You cannot connect blocks at this level. At simulation, connectivity is automatically
      | determined, based on the active variant and port name matching.
  Vbattery : Inport
  Throttle : Inport  Port=2
  envData : Inport  Port=3
  plantData : Inport  Port=4
  mappedMotor_1 : Subsystem  VariantControl=mappedMotors==1
  noMappedMotor_1 : Subsystem  VariantControl=mappedMotors~=1
  Im : Outport
  Thrust : Outport  Port=2
  Thrust_moment : Outport  Port=3

== system mainV02_33/LIBIS Plant/Propulsion/Variant_Motor_2 ==
  note: 1) Add Subsystem or Model blocks as valid variant choices.
      | 2) You cannot connect blocks at this level. At simulation, connectivity is automatically
      | determined, based on the active variant and port name matching.
  Vbattery : Inport
  Throttle : Inport  Port=2
  envData : Inport  Port=3
  plantData : Inport  Port=4
  mappedMotor_2 : Subsystem  VariantControl=mappedMotors==1
  noMappedMotor_2 : Subsystem  VariantControl=mappedMotors~=1
  Im : Outport
  Thrust : Outport  Port=2
  Thrust_moment : Outport  Port=3

== system mainV02_33/LIBIS Plant/Propulsion/Variant_Motor_3 ==
  note: 1) Add Subsystem or Model blocks as valid variant choices.
      | 2) You cannot connect blocks at this level. At simulation, connectivity is automatically
      | determined, based on the active variant and port name matching.
  Vbattery : Inport
  Throttle : Inport  Port=2
  envData : Inport  Port=3
  plantData : Inport  Port=4
  mappedMotor_3 : Subsystem  VariantControl=mappedMotors==1
  noMappedMotor_3 : Subsystem  VariantControl=mappedMotors~=1
  Im : Outport
  Thrust : Outport  Port=2
  Thrust_moment : Outport  Port=3

== system mainV02_33/LIBIS Plant/Propulsion/Variant_Motor_4 ==
  note: 1) Add Subsystem or Model blocks as valid variant choices.
      | 2) You cannot connect blocks at this level. At simulation, connectivity is automatically
      | determined, based on the active variant and port name matching.
  Vbattery : Inport
  Throttle : Inport  Port=2
  envData : Inport  Port=3
  plantData : Inport  Port=4
  mappedMotor_4 : Subsystem  VariantControl=mappedMotors==1
  noMappedMotor_4 : Subsystem  VariantControl=mappedMotors~=1
  Im : Outport
  Thrust : Outport  Port=2
  Thrust_moment : Outport  Port=3

== system mainV02_33/LIBIS Plant/Propulsion/Variant_Motor_5 ==
  note: 1) Add Subsystem or Model blocks as valid variant choices.
      | 2) You cannot connect blocks at this level. At simulation, connectivity is automatically
      | determined, based on the active variant and port name matching.
  Vbattery : Inport
  Throttle : Inport  Port=2
  envData : Inport  Port=3
  plantData : Inport  Port=4
  mappedMotor_5 : Subsystem  VariantControl=mappedMotors==1
  noMappedMotor_5 : Subsystem  VariantControl=mappedMotors~=1
  Im : Outport
  Thrust : Outport  Port=2
  Thrust_moment : Outport  Port=3

== system mainV02_33/LIBIS Plant/Subsystem/calc alpha_dot ==
  q : Inport
  alpha,beta : Inport  Port=2
  Ab : Inport  Port=3
  Vw : Inport  Port=4
  Direction Cosine Matrix Body to Wind : aerolibtransform2/Direction Cosine Matrix Body to Wind
  Product1 : Product  Multiplication=Matrix(*)  SaturateOnIntegerOverflow=on  InputSameDT=on  OutDataTypeStr=Inherit: Same as first input
  Product2 : Product  Inputs=*/  SaturateOnIntegerOverflow=on  InputSameDT=on  OutDataTypeStr=Inherit: Same as first input
  Selector2 : Selector  IndexMode=Zero-based  InputPortWidth=3  IndexOptions=Index vector (dialog)  Indices=2  OutputSizes=1
  Selector3 : Selector  IndexMode=Zero-based  InputPortWidth=3  IndexOptions=Index vector (dialog)  Indices=0  OutputSizes=1
  Sum : Sum  Inputs=++|
  Transpose1 : Math  Operator=transpose  SaturateOnIntegerOverflow=on
  alpha_dot : Outport
  wires:
  Direction Cosine Matrix Body to Wind/1 -> Transpose1/1
  Transpose1/1 -> Product1/1
  Product1/1 -> Selector2/1
  Selector2/1 -> Product2/1
  Selector3/1 -> Product2/2
  Product2/1 -> Sum/2
  alpha,beta/1 -> Direction Cosine Matrix Body to Wind/1
  q/1 -> Sum/1
  Sum/1 -> alpha_dot/1
  Ab/1 -> Product1/2
  Vw/1 -> Selector3/1

== system mainV02_33/LIBIS Plant/alpha_dot, beta_dot/Subsystem ==
  beta : Inport  Unit=rad
  alpha : Inport  Port=2  Unit=rad
  V_body : Inport  Port=3  Unit=meter/s
  Omega_body : Inport  Port=4  Unit=rad/s
  Accel_body : Inport  Port=5  Unit=m/s^2
  Constant11 : Constant  Value=0
  Direction Cosine Matrix Body to Wind : aerolibtransform2/Direction Cosine Matrix Body to Wind
  Mux4 : Mux  Inputs=2
  Product1 : Product  Multiplication=Matrix(*)  SaturateOnIntegerOverflow=on  InputSameDT=on  OutDataTypeStr=Inherit: Same as first input
  Selector : Selector  InputPortWidth=3  IndexOptions=Index vector (dialog)  Indices=[2]  OutputSizes=1
  calc alpha_dot : Subsystem
  alpha_dot : Outport  Unit=rad/s
  beta_dot : Outport  Port=2
  wires:
  Direction Cosine Matrix Body to Wind/1 -> Product1/1
  Product1/1 -> calc alpha_dot/4(Vw)
  Mux4/1 -> Direction Cosine Matrix Body to Wind/1, calc alpha_dot/2(alpha,beta)
  Constant11/1 -> beta_dot/1  "beta_dot"
  alpha/1 -> Mux4/1
  Omega_body/1 -> Selector/1
  V_body/1 -> Product1/2
  Accel_body/1 -> calc alpha_dot/3(Ab)
  beta/1 -> Mux4/2
  calc alpha_dot/1(alpha_dot) -> alpha_dot/1
  Selector/1 -> calc alpha_dot/1(q)  "q"

== system mainV02_33/Sensors (Feedthrough)/IMU/Calculate DCM & Euler Angles ==
  "p q r " : Inport
  Rotation Angles to Direction Cosine Matrix : aerolibtransform2/Rotation Angles to Direction Cosine Matrix  rotationOrder=ZYX
  Selector : Selector  InputPortWidth=3  IndexOptions=Index vector (dialog)  Indices=[3 2 1]  OutputSizes=1
  phi theta psi : Integrator  InitialCondition=[initialValues.roll0 initialValues.pitch0 initialValues.yaw0]
  phidot thetadot psidot : aerolib6dofsys/DCM & Euler Angles (Euler)/phidot thetadot psidot
  DCMMeas : Outport
  EulerMeas : Outport  Port=2
  wires:
  Selector/1 -> Rotation Angles to Direction Cosine Matrix/1
  phi theta psi/1 -> EulerMeas/1, Selector/1, phidot thetadot psidot/2
  phidot thetadot psidot/1 -> phi theta psi/1
  "p q r "/1 -> phidot thetadot psidot/1
  Rotation Angles to Direction Cosine Matrix/1 -> DCMMeas/1

== system mainV02_33/Visualization/Euler to VR/Axis Angle Vector ==
  e0 : Inport
  2 : Gain  Gain=2  SaturateOnIntegerOverflow=on  OutDataTypeStr=Inherit: Same as input  ParamDataTypeStr=Inherit: Same as input
  Concatenate : Concatenate
  Constant : Constant  Value=[0 0 0]
  Demux : Demux  Outputs=[1 3 ]
  Product : Product  Inputs=*/  SaturateOnIntegerOverflow=on  InputSameDT=on  OutDataTypeStr=Inherit: Same as first input
  Switch : Switch  Criteria=u2 > Threshold
  Trigonometric Function : Trigonometry
  Trigonometric Function2 : Trigonometry  Operator=acos
  e0_norm : Outport
  wires:
  Demux/1 -> Trigonometric Function2/1
  Demux/2 -> Product/1
  Concatenate/1 -> e0_norm/1
  2/1 -> Concatenate/2
  Trigonometric Function/1 -> Switch/2, Product/2
  Trigonometric Function2/1 -> Trigonometric Function/1, 2/1
  e0/1 -> Demux/1
  Switch/1 -> Concatenate/1
  Product/1 -> Switch/1
  Constant/1 -> Switch/3

== system mainV02_33/Visualization/Euler to VR/Quaternion Normalization ==
  e0 : Inport
  1/2 : Gain  Gain=1/2  SaturateOnIntegerOverflow=on  OutDataTypeStr=Inherit: Same as input  ParamDataTypeStr=Inherit: Same as input
  Concatenate : Concatenate
  Demux : Demux  Outputs=[1 3]
  Product : Product  SaturateOnIntegerOverflow=on  InputSameDT=on  OutDataTypeStr=Inherit: Same as first input
  Trigonometric Function : Trigonometry
  Trigonometric Function1 : Trigonometry  Operator=cos
  e0_norm : Outport
  wires:
  Trigonometric Function1/1 -> Concatenate/1
  Demux/2 -> Product/2
  Demux/1 -> 1/2/1
  Concatenate/1 -> e0_norm/1
  Product/1 -> Concatenate/2
  Trigonometric Function/1 -> Product/1
  1/2/1 -> Trigonometric Function1/1, Trigonometric Function/1
  e0/1 -> Demux/1

== system mainV02_33/Visualization/Euler to VR/Quaternion Normalization1 ==
  e0 : Inport
  1/2 : Gain  Gain=1/2  SaturateOnIntegerOverflow=on  OutDataTypeStr=Inherit: Same as input  ParamDataTypeStr=Inherit: Same as input
  Concatenate : Concatenate
  Demux : Demux  Outputs=[1 3]
  Product : Product  SaturateOnIntegerOverflow=on  InputSameDT=on  OutDataTypeStr=Inherit: Same as first input
  Trigonometric Function : Trigonometry
  Trigonometric Function1 : Trigonometry  Operator=cos
  e0_norm : Outport
  wires:
  e0/1 -> Demux/1
  1/2/1 -> Trigonometric Function/1, Trigonometric Function1/1
  Trigonometric Function/1 -> Product/1
  Product/1 -> Concatenate/2
  Concatenate/1 -> e0_norm/1
  Demux/1 -> 1/2/1
  Demux/2 -> Product/2
  Trigonometric Function1/1 -> Concatenate/1

== system mainV02_33/Visualization/Euler to VR/Quaternion Normalization2 ==
  e0 : Inport
  1/2 : Gain  Gain=1/2  SaturateOnIntegerOverflow=on  OutDataTypeStr=Inherit: Same as input  ParamDataTypeStr=Inherit: Same as input
  Concatenate : Concatenate
  Demux : Demux  Outputs=[1 3]
  Product : Product  SaturateOnIntegerOverflow=on  InputSameDT=on  OutDataTypeStr=Inherit: Same as first input
  Trigonometric Function : Trigonometry
  Trigonometric Function1 : Trigonometry  Operator=cos
  e0_norm : Outport
  wires:
  Trigonometric Function1/1 -> Concatenate/1
  Demux/2 -> Product/2
  Demux/1 -> 1/2/1
  Concatenate/1 -> e0_norm/1
  Product/1 -> Concatenate/2
  Trigonometric Function/1 -> Product/1
  1/2/1 -> Trigonometric Function1/1, Trigonometric Function/1
  e0/1 -> Demux/1

== system mainV02_33/Visualization/Subsystem/Flightpath Angle ==
  Ve : Inport
  Constant : Constant  Value=eps
  Sum2 : Sum  Inputs=+  SaturateOnIntegerOverflow=on  InputSameDT=on  OutDataTypeStr=Inherit: Same as first input
  Switch : Switch  Criteria=u2 > Threshold
  product : Product  SaturateOnIntegerOverflow=on  InputSameDT=on  OutDataTypeStr=Inherit: Same as first input
  product1 : Product  Inputs=/*  SaturateOnIntegerOverflow=on  InputSameDT=on  OutDataTypeStr=Inherit: Same as first input
  rad-->deg4 : Gain  Gain=-1  SaturateOnIntegerOverflow=on  OutDataTypeStr=Inherit: Same as input  ParamDataTypeStr=Inherit: Same as input
  tangent : Trigonometry  Operator=atan
  u,v : Selector  IndexMode=Zero-based  InputPortWidth=3  IndexOptions=Index vector (dialog)  Indices=[0 1]  OutputSizes=1
  v : Sqrt  SaturateOnIntegerOverflow=on
  w : Selector  IndexMode=Zero-based  InputPortWidth=3  IndexOptions=Index vector (dialog)  Indices=2  OutputSizes=1
  gamma : Outport
  wires:
  Ve/1 -> w/1, u,v/1
  product/1 -> Sum2/1
  Sum2/1 -> v/1
  product1/1 -> tangent/1
  u,v/1 -> product/2, product/1
  w/1 -> rad-->deg4/1
  v/1 -> Switch/2, product1/1
  rad-->deg4/1 -> product1/2
  tangent/1 -> Switch/1
  Constant/1 -> Switch/3
  Switch/1 -> gamma/1

== system mainV02_33/LIBIS Plant/Propulsion/Variant_Motor_1/mappedMotor_1 ==
  Vbattery : Inport
  Throttle : Inport  Port=2
  envData : Inport  Port=3
  plantData : Inport  Port=4
  3x3 Cross Product : aerolibutil/3x3 Cross Product
  Bus Selector : BusSelector  OutputSignals=V_body,CG,LLA.Altitude_m
  Bus Selector1 : BusSelector  OutputSignals=windVelocity
  Constant{1..4} (4 alike) : Constant  Value=0
  ESC_1 : Subsystem
  Motor and Propeller Coupling_1 : Subsystem
  Mux : Mux  Inputs=3
  Mux1 : Mux  Inputs=3
  Selector1 : Selector  InputPortWidth=3  IndexOptions=Index vector (dialog)  Indices=[1]  OutputSizes=1
  Selector2 : Selector  InputPortWidth=3  IndexOptions=Index vector (dialog)  Indices=[1]  OutputSizes=1
  Sum : Sum  Inputs=|+-
  Sum1 : Sum  Inputs=+-|
  Sum2 : Sum  Inputs=|++
  Terminator : Terminator
  Torque : Subsystem
  "motor2 position " : Constant  Value=LD.Propulsion.motor1.Position
  Im : Outport
  Thrust : Outport  Port=2
  Thrust_moment : Outport  Port=3
  wires:
  Vbattery/1 -> ESC_1/1(V_battery)
  ESC_1/1(V_ESC) -> Motor and Propeller Coupling_1/1(Voltage)  "V_ESC"
  Mux/1 -> Thrust/1, 3x3 Cross Product/2  "Thrust_vector"
  Throttle/1 -> ESC_1/2(Throttle)
  Constant1/1 -> Mux/2
  Sum1/1 -> 3x3 Cross Product/1  "arm"
  Motor and Propeller Coupling_1/3(Current) -> Im/1
  Bus Selector/2 -> [CG]  "<CG>"
  Bus Selector/3 -> [Altitude]  "<Altitude_m>"
  Bus Selector1/1 -> [V_wind]  "<windVelocity>"
  [CG] -> Sum1/2
  Selector2/1 -> Sum/1
  Selector1/1 -> Sum/2
  plantData/1 -> Bus Selector/1
  [V_body] -> Selector2/1
  Motor and Propeller Coupling_1/1(Thrust) -> Mux/1  "Thrust_scalar"
  [Altitude] -> Motor and Propeller Coupling_1/2(Height)
  "motor2 position "/1 -> Sum1/1
  [V_wind] -> Selector1/1
  Constant2/1 -> Mux/3
  Bus Selector/1 -> [V_body]  "<V_body>"
  envData/1 -> Bus Selector1/1
  Motor and Propeller Coupling_1/2(Power) -> Terminator/1
  Sum/1 -> Torque/2(Vflight), Motor and Propeller Coupling_1/3(Vflight)
  Mux1/1 -> Sum2/2  "Torque_vector"
  Constant3/1 -> Mux1/2
  Sum2/1 -> Thrust_moment/1
  3x3 Cross Product/1 -> Sum2/1
  Motor and Propeller Coupling_1/4(RPM) -> Torque/1(RPM)  "RPM"
  Constant4/1 -> Mux1/3
  Torque/1(Torque) -> Mux1/1
